simulink subsystem "AAI_mode"  (R2022a)
settings: Solver=VariableStepAuto  StartTime=0.0  StopTime=10.0  RelTol=1e-3
settings Model: Creator=ivanl  LastModifiedBy=ivanl

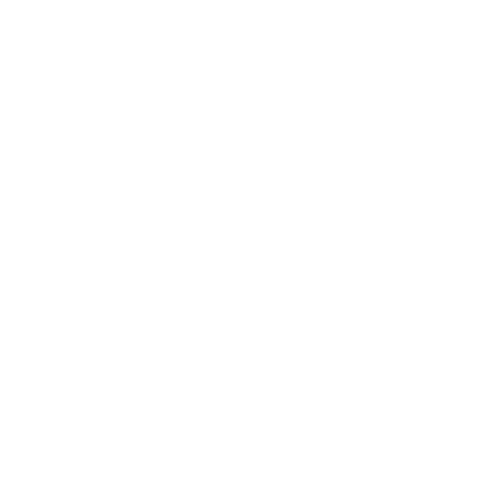
[thumbnail: Simulink's stored preview of the top-level diagram]
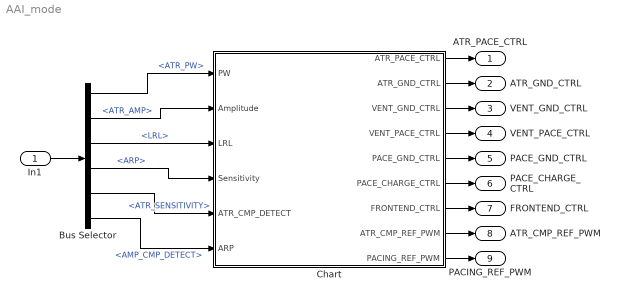
== system AAI_mode ==
  In1 : Inport
  Bus Selector : BusSelector  OutputSignals=ATR_PW,ATR_AMP,LRL,ARP,ATR_SENSITIVITY,AMP_CMP_DETECT
  Chart : Stateflow chart  TreatAsAtomicUnit=on
      settings: PortSchema="{\"entries\":[{\"content\":{\"sides\":[{\"content\":{\"connectorIds\":[\"In1\",\"In2\",\"In3\",\"In4\",\"In5\",\"In6\"]},\"type\":\"ConnectorPlacement.EquallySpacedRectSide\",\"uuid\":\"2dca410f-8f43-416b-b245-db6a1c9e2101\"},{\"content\":{\"connectorIds\":[\"Out2\",\"Out1\",\"Out4\",\"Out5\",\"Out6\",\"Out3\",\"Out8\",\"Out9\",\"Out7\"],\"side\":\"RIGHT\"},\"type\":\"ConnectorPlacement.EquallySpacedRectSide\",\"uuid\":\"30508f3d-7d2b-4c80-aa19-382c3c260e83\"},{\"content\":{\"connectorIds\":[],\"side\":\"TOP\"},\"type\":\"ConnectorPlacement.EquallySpacedRectSide\",\"uuid\":\"0cf054d9-a9d5-4fcc-8b60-c098224d8790\"}]},\"type\":\"ConnectorPlacement.EquallySpacedConnector\",\"uuid\":\"125de75b-c166-48e2-8d91-77ead1c82200\"}],\"packageUris\":[\"http://schema.mathworks.com/mf0/Connector/R2020b\"],\"version\":\"1.0\"}"
  ATR_PACE_CTRL : Outport
  ATR_GND_CTRL : Outport  Port=2
  VENT_GND_CTRL : Outport  Port=3
  VENT_PACE_CTRL : Outport  Port=4
  PACE_GND_CTRL : Outport  Port=5
  PACE_CHARGE_CTRL : Outport  Port=6
  FRONTEND_CTRL : Outport  Port=7
  ATR_CMP_REF_PWM : Outport  Port=8
  PACING_REF_PWM : Outport  Port=9
  wires:
  In1/1 -> Bus Selector/1
  Bus Selector/5 -> Chart/5(ATR_CMP_DETECT)  "<ATR_SENSITIVITY>"
  Bus Selector/6 -> Chart/6(ARP)  "<AMP_CMP_DETECT>"
  Bus Selector/1 -> Chart/1(PW)  "<ATR_PW>"
  Bus Selector/2 -> Chart/2(Amplitude)  "<ATR_AMP>"
  Bus Selector/3 -> Chart/3(LRL)  "<LRL>"
  Bus Selector/4 -> Chart/4(Sensitivity)  "<ARP>"
  Chart/2(ATR_PACE_CTRL) -> ATR_PACE_CTRL/1
  Chart/7(PACING_REF_PWM) -> PACING_REF_PWM/1
  Chart/9(ATR_CMP_REF_PWM) -> ATR_CMP_REF_PWM/1
  Chart/8(FRONTEND_CTRL) -> FRONTEND_CTRL/1
  Chart/3(PACE_CHARGE_CTRL) -> PACE_CHARGE_CTRL/1
  Chart/6(PACE_GND_CTRL) -> PACE_GND_CTRL/1
  Chart/5(VENT_PACE_CTRL) -> VENT_PACE_CTRL/1
  Chart/4(VENT_GND_CTRL) -> VENT_GND_CTRL/1
  Chart/1(ATR_GND_CTRL) -> ATR_GND_CTRL/1

== stateflow chart AAI_mode/Chart ==
  state AAI_Charging_C22
    entry:
    VENT_PACE_CTRL = false;
    ATR_PACE_CTRL = false;
    PACE_CHARGE_CTRL = true;
    PACING_REF_PWM = Amplitude * 20;
    PACE_GND_CTRL= true;
    VENT_GND_CTRL = false;
    ATR_GND_CTRL = true;
  state AAI_Pacing
    entry:
    PACE_CHARGE_CTRL = false;
    PACE_GND_CTRL = true;
    VENT_PACE_CTRL = false;
    VENT_GND_CTRL = false;
    ATR_GND_CTRL = false;
    ATR_PACE_CTRL = true;
  state AAI_Sensing
    entry:
    FRONTEND_CTRL = true;
    ATR_CMP_REF_PWM = (Sensitivity)*30;
    exit:
    FRONTEND_CTRL = false;
  (default) -> AAI_Charging_C22
  AAI_Pacing -> AAI_Charging_C22 : after(PW, msec)
  AAI_Sensing -> AAI_Pacing [order 2] : after(((60000/LRL) - ARP), msec)
  AAI_Sensing -> AAI_Charging_C22 [order 1] : [ATR_CMP_DETECT == true]
  AAI_Charging_C22 -> AAI_Sensing : after(ARP, msec)
  data: ATR_GND_CTRL output boolean; ATR_PACE_CTRL output boolean; PACE_CHARGE_CTRL output boolean; VENT_GND_CTRL output boolean; VENT_PACE_CTRL output boolean; PACE_GND_CTRL output boolean; PW input double; Amplitude input double; LRL input double; PACING_REF_PWM output double; Sensitivity input double; FRONTEND_CTRL output boolean; ATR_CMP_DETECT input boolean; ARP input double; ATR_CMP_REF_PWM output double
